simulink model "servo_control_with_observer"  (R2017a)
settings: Solver=VariableStepAuto  StartTime=0.0  StopTime=25  RelTol=1e-3
values from neighbouring files (symbols this model uses):
  A = [-8.8487+(a-b)/5 -0.0399 -5.55+(c+d)/10 3.5846 ... (first row only)    [initialize.m]
  B = [0.0564+b/(10+c) 0.0319 ... (first row only)    [initialize.m]
  C = [-3.2988 -2.1932+(10*c+d)/(100+5*a) 0.037 -0.0109 ... (first row only)    [initialize.m]
  K1 = K_LQR(:,1:4)    [MIMO_servo_control_with_observer.m]    (also in MIMO_servo_control_without_observer.m; last_task.m)
  K2 = K_LQR(:,5:6)    [MIMO_servo_control_with_observer.m]    (also in MIMO_servo_control_without_observer.m; last_task.m)
  L = transpose(K)    [MIMO_servo_control_with_observer.m]    (also in full_order_observer.m)
settings Model: Creator=lenovo  LastModifiedBy=lenovo

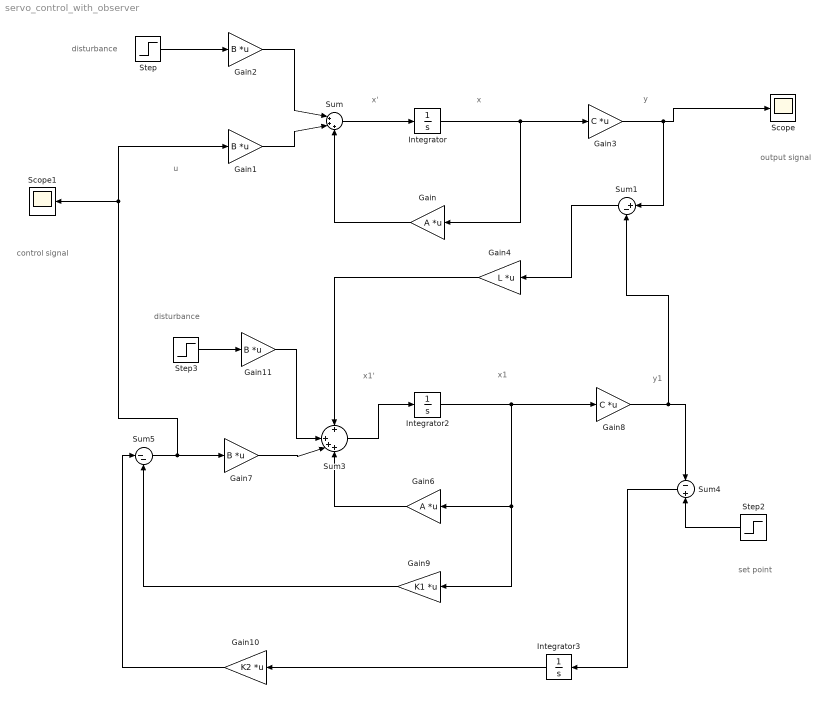
== system servo_control_with_observer ==
  note: disturbance
  note: control signal
  note: set point
  note: output signal
  note: u
  note: y1
  note: x1'
  note: x1
  note: x'
  note: x
  note: y
  note: disturbance
  Gain : Gain  Gain=A  Multiplication=Matrix(K*u)
  Gain{1..2,7,11} (4 alike) : Gain  Gain=B  Multiplication=Matrix(K*u)
  Gain10 : Gain  Gain=K2  Multiplication=Matrix(K*u)
  Gain3 : Gain  Gain=C  Multiplication=Matrix(K*u)
  Gain4 : Gain  Gain=L  Multiplication=Matrix(K*u)
  Gain6 : Gain  Gain=A  Multiplication=Matrix(K*u)
  Gain8 : Gain  Gain=C  Multiplication=Matrix(K*u)
  Gain9 : Gain  Gain=K1  Multiplication=Matrix(K*u)
  Integrator : Integrator  InitialCondition=[0.5;-0.1;0.3;-0.8]
  Integrator2 : Integrator
  Integrator3 : Integrator
  Scope : Scope
  Scope1 : Scope
  Step : Step  Time=10  Before=[0;0]  After=[0.3;0.2]  SampleTime=0  VectorParams1D=off
  Step2 : Step  Time=0  Before=[0;0]  After=[0.4;0.8]  SampleTime=0  VectorParams1D=off
  Step3 : Step  Time=10  Before=[0;0]  After=[0.3;0.2]  SampleTime=0  VectorParams1D=off
  Sum : Sum  Inputs=|+++
  Sum1 : Sum  Inputs=|+-
  Sum3 : Sum  Inputs=+|+++
  Sum4 : Sum  Inputs=-|+
  Sum5 : Sum  Inputs=|--
  wires:
  Step/1 -> Gain2/1
  Gain2/1 -> Sum/1
  Sum/1 -> Integrator/1
  Integrator/1 -> Gain3/1, Gain/1
  Gain3/1 -> Sum1/1, Scope/1
  Gain/1 -> Sum/3
  Gain1/1 -> Sum/2
  Integrator2/1 -> Gain8/1, Gain9/1, Gain6/1
  Step2/1 -> Sum4/2
  Gain8/1 -> Sum1/2, Sum4/1
  Sum4/1 -> Integrator3/1
  Integrator3/1 -> Gain10/1
  Gain10/1 -> Sum5/1
  Gain9/1 -> Sum5/2
  Step3/1 -> Gain11/1
  Gain6/1 -> Sum3/4
  Gain7/1 -> Sum3/3
  Gain11/1 -> Sum3/2
  Sum1/1 -> Gain4/1
  Gain4/1 -> Sum3/1
  Sum3/1 -> Integrator2/1
  Sum5/1 -> Gain1/1, Scope1/1, Gain7/1
